simulink model "sampleModel1477"  (R2023a)
settings: Solver=VariableStepAuto  StartTime=0.0  StopTime=10.0  RelTol=1e-3
libraries: simulink x2, hdlsllib x2
settings Model: Creator=user1  LastModifiedBy=user1

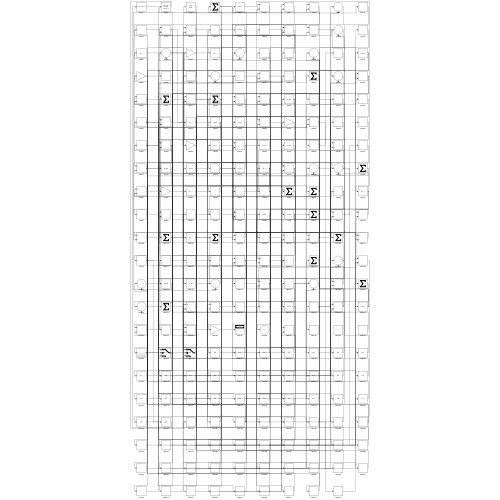
[thumbnail: Simulink's stored preview of the top-level diagram]
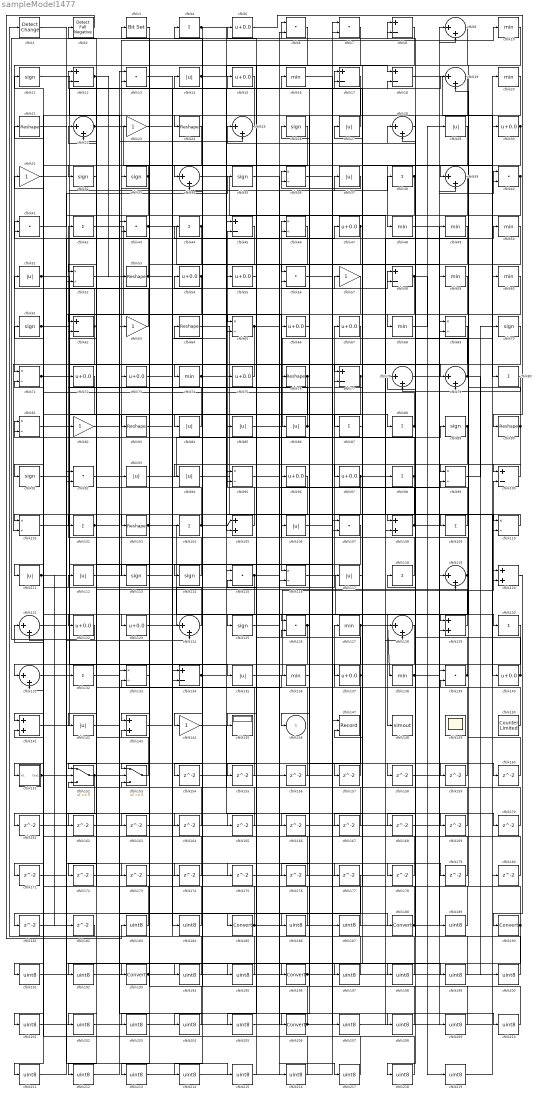
== system sampleModel1477 ==
  cfblk1 : simulink/Logic and Bit Operations/Detect Change  vinit=0  OutDataTypeStr=boolean
      settings: LibrarySourceBlock=|
      | hdlsllib/Logic and Bit
      | Operations/Detect
      | Change
  cfblk{10,16,20,48..50,59..60,68,74,127,136,138} (13 alike) : MinMax
  cfblk{8,12,17..18,45,58,62,77,100,134} (10 alike) : Sum  Inputs=+-
  cfblk{36,46,52,65,69,71,81,95,99,101,110,116,133} (13 alike) : Product  Inputs=*/  RndMeth=Zero  SaturateOnIntegerOverflow=on
  cfblk{4,38,42,44,80,87..88,98,102,104,109,118,130,132} (14 alike) : Sum  Inputs=+
  cfblk{21,24,53,64,76,83,90,103} (8 alike) : Reshape
  cfblk{105,108,120,129,141,143} (6 alike) : Sum
  cfblk{14,27,29,37,51,84..86,93..94,106,111..112,117,135,142} (16 alike) : Abs  SaturateOnIntegerOverflow=off
  cfblk{6..7,13,40..41,43,56,92,107,115,126,139} (12 alike) : DotProduct  OutDataTypeStr=Inherit: Inherit via internal rule
  cfblk{11,26,32..33,35,61,70,89,91,113..114,125} (12 alike) : Signum
  cfblk{9,19,22,25,28,34,39,78..79,119,121,124,128,131} (14 alike) : Sum  Inputs=|++
  cfblk{5,15,30,47,54..55,66..67,72..73,75,96..97,122..123,137,140} (17 alike) : Bias  Bias=0.0  SaturateOnIntegerOverflow=off
  cfblk{23,31,57,63,82,144} (6 alike) : Gain
  cfblk145 : Display
  cfblk147 : Record  FileSettingsInternal="{\"entries\":[{\"content\":{\"excelSettings\":{\"content\":{},\"type\":\"Streamout.ExcelSettings\"}},\"type\":\"Streamout.FileSettingStorage\",\"uuid\":\"\"}],\"packageUris\":[\"http:\\/\\/schema.mathworks.com\\/mf0\\/streamout_blocks\\/R2020a\"],\"version\":\"1.0\"}"  Layout=[1 1]  SignalsInternal="{\"entries\":[{\"content\":{\"signals\":[{\"content\":{\"blockPath\":[],\"dimensions\":[1],\"domain\":\"\",\"lineColor\":\"#a2142f\",\"plots\":[1],\"port\":1,\"signalID\":1073,\"signalName\":\"XY Graph:1\"},\"type\":\"RecordBlkView.Signal\",\"uuid\":\"\"},{\"content\":{\"blockPath\":[],\"dimensions\":[1],\"domain\":\"\",\"lineColor\":\"#139fff\",\"plots\":[1],\"port\":2,\"signalID\":1076,\"signalName\":\"XY Graph:2\"},\"type\":\"RecordBlkView.Signal\",\"uuid\":\"\"}]},\"type\":\"RecordBlkView.InputSignals\",\"uuid\":\"\"}],\"packageUris\":[\"http:\\/\\/schema.mathworks.com\\/mf0\\/streamout_blocks\\/R2020a\"],\"version\":\"1.0\"}"  VisualizationBindings="{\"xyplotplugin\":{\"info\":[{\"series\":[{\"bindingParametersList\":[{\"parameter\":\"X-Axis\",\"signalID\":1073,\"signalName\":\"XY Graph:1\"},{\"parameter\":\"Y-Axis\",\"signalID\":1076,\"signalName\":\"XY Graph:2\"}],\"seriesID\":12696}],\"subplotID\":1}]}}"  CompatibilityTag=XY  st=-1
  cfblk148 : ToWorkspace  VariableName=simout  SaveFormat=Timeseries  SampleTime=-1
  cfblk149 : Scope
      settings: Floating=on
  cfblk150 : hdlsllib/Sources/Counter Limited  uplimit=7  tsamp=-1
  cfblk151 : Subsystem
      settings: LibrarySourceBlock=|
      | hdlsllib/Ports &
      | Subsystems/Subsystem
  cfblk152 : Switch  SaturateOnIntegerOverflow=off  InputSameDT=off
  cfblk153 : Switch  SaturateOnIntegerOverflow=off  InputSameDT=off
  cfblk{154..182} (29 alike) : Delay  SampleTime=1
  cfblk{183..184,186..187,189,191..192,194..195,197..205,207..219} (31 alike) : DataTypeConversion  OutDataTypeStr=uint8  SaturateOnIntegerOverflow=off  RndMeth=Floor
  cfblk{185,188,190,193,196,206} (6 alike) : DataTypeConversion  SaturateOnIntegerOverflow=off  RndMeth=Floor
  cfblk2 : hdlsllib/Logic and Bit Operations/Detect Fall Negative  vinit=0  OutDataTypeStr=boolean
  cfblk3 : simulink/Logic and Bit Operations/Bit Set  iBit=0
      settings: LibrarySourceBlock=|
      | hdlsllib/Logic and Bit
      | Operations/Bit Set
  cfblk146 : Outport  VectorParamsAs1DForOutWhenUnconnected=off
  wires:
  cfblk123/1 -> cfblk67/1
  cfblk99/1 -> cfblk70/1
  cfblk68/1 -> cfblk29/1
  cfblk112/1 -> cfblk10/1
  cfblk75/1 -> cfblk74/1
  cfblk86/1 -> cfblk73/1, cfblk146/1
  cfblk90/1 -> cfblk100/1, cfblk44/1, cfblk176/1
  cfblk77/1 -> cfblk154/1, cfblk186/1
  cfblk122/1 -> cfblk6/1
  cfblk59/1 -> cfblk116/1
  cfblk73/1 -> cfblk58/1
  cfblk60/1 -> cfblk206/1
  cfblk46/1 -> cfblk153/1
  cfblk119/1 -> cfblk46/1, cfblk141/1
  cfblk22/1 -> cfblk39/1, cfblk179/1
  cfblk109/1 -> cfblk17/1
  cfblk118/1 -> cfblk14/1
  cfblk31/1 -> cfblk196/1
  cfblk5/1 -> cfblk90/1
  cfblk141/1 -> cfblk17/2
  cfblk133/1 -> cfblk193/1
  cfblk61/1 -> cfblk135/1, cfblk57/1
  cfblk51/1 -> cfblk88/1, cfblk173/1
  cfblk37/1 -> cfblk36/1
  cfblk38/1 -> cfblk77/1, cfblk62/1
  cfblk18/1 -> cfblk80/1
  cfblk135/1 -> cfblk100/2
  cfblk7/1 -> cfblk71/1
  cfblk115/1 -> cfblk99/2, cfblk155/1, cfblk192/1
  cfblk101/1 -> cfblk37/1
  cfblk110/1 -> cfblk101/1
  cfblk21/1 -> cfblk66/1
  cfblk54/1 -> cfblk122/1, cfblk213/1
  cfblk34/1 -> cfblk98/1
  cfblk10/1 -> cfblk129/1
  cfblk85/1 -> cfblk30/1
  cfblk150/1 -> cfblk127/1
  cfblk71/1 -> cfblk79/1, cfblk153/2
  cfblk152/1 -> cfblk136/1, cfblk211/1
  cfblk140/1 -> cfblk78/1, cfblk85/1
  cfblk25/1 -> cfblk24/1
  cfblk104/1 -> cfblk105/1, cfblk62/2
  cfblk82/1 -> cfblk188/1
  cfblk153/1 -> cfblk112/1
  cfblk65/1 -> cfblk152/1, cfblk177/1
  cfblk17/1 -> cfblk144/1
  cfblk116/1 -> cfblk148/1
  cfblk30/1 -> cfblk48/1, cfblk68/1
  cfblk11/1 -> cfblk63/1
  cfblk14/1 -> cfblk34/1, cfblk18/1
  cfblk64/1 -> cfblk106/1
  cfblk1/1 -> cfblk124/2
  cfblk105/1 -> cfblk45/2
  cfblk84/1 -> cfblk42/1
  cfblk12/1 -> cfblk142/1, cfblk53/1
  cfblk58/1 -> cfblk145/1, cfblk209/1
  cfblk100/1 -> cfblk99/1
  cfblk39/1 -> cfblk52/1
  cfblk27/1 -> cfblk12/1
  cfblk136/1 -> cfblk96/1
  cfblk36/1 -> cfblk109/1
  cfblk9/1 -> cfblk65/1
  cfblk127/1 -> cfblk138/1, cfblk50/1, cfblk195/1
  cfblk111/1 -> cfblk47/1, cfblk182/1
  cfblk117/1 -> cfblk27/1
  cfblk44/1 -> cfblk84/1, cfblk113/1
  cfblk19/1 -> cfblk126/1
  cfblk91/1 -> cfblk147/1
  cfblk45/1 -> cfblk83/1
  cfblk114/1 -> cfblk72/1
  cfblk63/1 -> cfblk21/1
  cfblk24/1 -> cfblk131/1
  cfblk134/1 -> cfblk19/1, cfblk4/1
  cfblk47/1 -> cfblk123/1, cfblk56/1
  cfblk67/1 -> cfblk152/2
  cfblk74/1 -> cfblk110/1, cfblk108/1
  cfblk94/1 -> cfblk140/1
  cfblk103/1 -> cfblk130/1, cfblk169/1
  cfblk139/1 -> cfblk118/1, cfblk25/1
  cfblk80/1 -> cfblk78/2
  cfblk42/1 -> cfblk75/1
  cfblk53/1 -> cfblk143/1, cfblk18/2, cfblk11/1
  cfblk62/1 -> cfblk101/2, cfblk41/1, cfblk91/1
  cfblk143/1 -> cfblk65/2
  cfblk137/1 -> cfblk55/1, cfblk166/1, cfblk167/1
  cfblk151/1(Out1) -> cfblk58/2, cfblk164/1
  cfblk129/1 -> cfblk22/2
  cfblk79/1 -> cfblk8/1, cfblk200/1
  cfblk124/1 -> cfblk81/1
  cfblk89/1 -> cfblk116/2, cfblk94/1
  cfblk43/1 -> cfblk119/1, cfblk87/1
  cfblk83/1 -> cfblk38/1
  cfblk70/1 -> cfblk103/1
  cfblk93/1 -> cfblk89/1
  cfblk52/1 -> cfblk104/1
  cfblk66/1 -> cfblk36/2
  cfblk108/1 -> cfblk95/1, cfblk40/1
  cfblk126/1 -> cfblk26/1, cfblk205/1
  cfblk81/1 -> cfblk7/2
  cfblk69/1 -> cfblk114/1
  cfblk138/1 -> cfblk9/1, cfblk9/2
  cfblk4/1 -> cfblk34/2, cfblk8/2, cfblk40/2
  cfblk29/1 -> cfblk137/1
  cfblk40/1 -> cfblk86/1, cfblk102/1
  cfblk120/1 -> cfblk190/1
  cfblk50/1 -> cfblk105/2
  cfblk76/1 -> cfblk171/1, cfblk172/1
  cfblk13/1 -> cfblk185/1
  cfblk8/1 -> cfblk97/1
  cfblk96/1 -> cfblk125/1
  cfblk6/1 -> cfblk95/2
  cfblk102/1 -> cfblk23/1, cfblk25/2
  cfblk48/1 -> cfblk69/2
  cfblk41/1 -> cfblk35/1
  cfblk98/1 -> cfblk41/2, cfblk194/1
  cfblk97/1 -> cfblk111/1, cfblk110/2, cfblk203/1
  cfblk72/1 -> cfblk151/1(In1)
  cfblk88/1 -> cfblk61/1, cfblk76/1
  cfblk33/1 -> cfblk32/1, cfblk3/1, cfblk92/2
  cfblk154/1 -> cfblk7/1
  cfblk155/1 -> cfblk45/1
  cfblk156/1 -> cfblk43/1
  cfblk95/1 -> cfblk157/1
  cfblk157/1 -> cfblk22/1
  cfblk142/1 -> cfblk158/1
  cfblk158/1 -> cfblk39/2
  cfblk92/1 -> cfblk159/1
  cfblk159/1 -> cfblk46/2
  cfblk106/1 -> cfblk160/1
  cfblk160/1 -> cfblk19/2
  cfblk15/1 -> cfblk161/1
  cfblk161/1 -> cfblk119/2
  cfblk32/1 -> cfblk162/1
  cfblk162/1 -> cfblk69/1
  cfblk3/1 -> cfblk163/1
  cfblk163/1 -> cfblk124/1
  cfblk164/1 -> cfblk152/3
  cfblk55/1 -> cfblk165/1
  cfblk165/1 -> cfblk115/1
  cfblk167/1 -> cfblk12/2
  cfblk130/1 -> cfblk168/1
  cfblk168/1 -> cfblk129/2
  cfblk169/1 -> cfblk143/2
  cfblk144/1 -> cfblk170/1
  cfblk170/1 -> cfblk79/2
  cfblk171/1 -> cfblk52/2
  cfblk172/1 -> cfblk134/2
  cfblk173/1 -> cfblk108/2
  cfblk131/1 -> cfblk174/1
  cfblk174/1 -> cfblk71/2
  cfblk113/1 -> cfblk175/1
  cfblk176/1 -> cfblk153/3
  cfblk35/1 -> cfblk178/1
  cfblk178/1 -> cfblk77/2
  cfblk179/1 -> cfblk81/2
  cfblk180/1 -> cfblk126/2
  cfblk26/1 -> cfblk181/1
  cfblk182/1 -> cfblk1/1
  cfblk2/1 -> cfblk183/1
  cfblk183/1 -> cfblk51/1
  cfblk23/1 -> cfblk184/1
  cfblk184/1 -> cfblk2/1
  cfblk185/1 -> cfblk141/2, cfblk139/1, cfblk131/2, cfblk115/2
  cfblk186/1 -> cfblk13/1
  cfblk166/1 -> cfblk187/1
  cfblk187/1 -> cfblk13/2
  cfblk188/1 -> cfblk56/2, cfblk219/1
  cfblk78/1 -> cfblk189/1
  cfblk189/1 -> cfblk82/1
  cfblk190/1 -> cfblk139/2, cfblk147/2, cfblk202/1
  cfblk177/1 -> cfblk191/1
  cfblk191/1 -> cfblk120/1
  cfblk192/1 -> cfblk120/2
  cfblk193/1 -> cfblk117/1, cfblk6/2
  cfblk194/1 -> cfblk133/1
  cfblk195/1 -> cfblk133/2
  cfblk196/1 -> cfblk180/1, cfblk59/1
  cfblk87/1 -> cfblk197/1
  cfblk197/1 -> cfblk31/1
  cfblk28/1 -> cfblk198/1
  cfblk198/1 -> cfblk134/1
  cfblk181/1 -> cfblk199/1
  cfblk199/1 -> cfblk28/1
  cfblk200/1 -> cfblk28/2
  cfblk128/1 -> cfblk201/1
  cfblk201/1 -> cfblk156/1
  cfblk202/1 -> cfblk128/1
  cfblk203/1 -> cfblk128/2
  cfblk49/1 -> cfblk204/1
  cfblk204/1 -> cfblk43/2
  cfblk205/1 -> cfblk49/1
  cfblk206/1 -> cfblk15/1, cfblk64/1
  cfblk56/1 -> cfblk207/1
  cfblk207/1 -> cfblk60/1
  cfblk16/1 -> cfblk208/1
  cfblk208/1 -> cfblk33/1
  cfblk209/1 -> cfblk16/1
  cfblk132/1 -> cfblk210/1
  cfblk210/1 -> cfblk54/1
  cfblk211/1 -> cfblk132/1
  cfblk107/1 -> cfblk212/1
  cfblk212/1 -> cfblk93/1
  cfblk213/1 -> cfblk107/1
  cfblk57/1 -> cfblk214/1
  cfblk214/1 -> cfblk107/2
  cfblk121/1 -> cfblk215/1
  cfblk215/1 -> cfblk5/1
  cfblk125/1 -> cfblk216/1
  cfblk216/1 -> cfblk121/1
  cfblk175/1 -> cfblk217/1
  cfblk217/1 -> cfblk121/2
  cfblk20/1 -> cfblk218/1
  cfblk218/1 -> cfblk92/1
  cfblk219/1 -> cfblk20/1

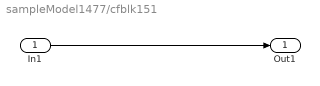
== system sampleModel1477/cfblk151 ==
  In1 : Inport
  Out1 : Outport
  wires:
  In1/1 -> Out1/1
